simulink model "pathFollowingRetta_Lyap"  (R2022b)
settings: Solver=VariableStepAuto  StartTime=0.0  StopTime=10.0  RelTol=1e-3
undefined symbols (not defined in the file): q0
settings Model: Creator=Lorenzo Albertini  LastModifiedBy=Lorenzo Albertini

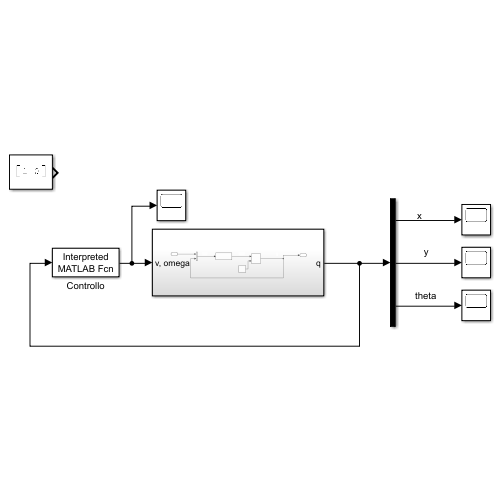
[thumbnail: Simulink's stored preview of the top-level diagram]
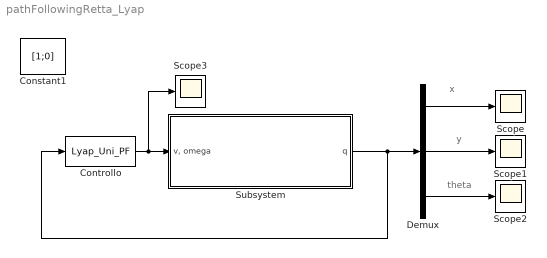
== system pathFollowingRetta_Lyap ==
  note: theta
  note: y
  note: x
  Constant1 : Constant  Value=[1;0]
  Controllo : MATLABFcn  MATLABFcn=Lyap_Uni_PF
  Demux : Demux  Outputs=3
  Scope{,1..3} (4 alike) : Scope
  Subsystem : Subsystem
  wires:
  Subsystem/1(q) -> Demux/1, Controllo/1
  Controllo/1 -> Scope3/1, Subsystem/1("v, omega")
  Demux/1 -> Scope/1
  Demux/3 -> Scope2/1
  Demux/2 -> Scope1/1

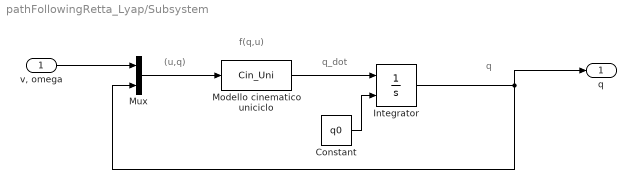
== system pathFollowingRetta_Lyap/Subsystem ==
  note: (u,q)
  note: q
  note: q_dot
  note: f(q,u)
  "v, omega" : Inport
  Constant : Constant  Value=q0
  Integrator : Integrator  InitialConditionSource=external
  Modello cinematico uniciclo : MATLABFcn  MATLABFcn=Cin_Uni
  Mux : Mux  Inputs=2
  q : Outport
  wires:
  Integrator/1 -> q/1, Mux/2
  Modello cinematico uniciclo/1 -> Integrator/1
  "v, omega"/1 -> Mux/1
  Mux/1 -> Modello cinematico uniciclo/1
  Constant/1 -> Integrator/2
